simulink model "bcccc"  (Simulink 7.4)
settings: Solver=ode1  StartTime=0.0  StopTime=1000  FixedStep=T  RelTol=1e-3  AbsTol=1e-6
values from neighbouring files (symbols this model uses):
  calibParams = [469.5 7.95034094731e-05 741.8 8.4355330608e-05 2167.3 0.000136518771331]    [bcc.mat]    (also in calibParams.mat = [471.3 8.26262433661e-05 786 8.69187309865e-05 2173.5 0.0001)
  T = 0.5    [bcc.mat]    (also in hydrostart.m = 0.25)
libraries: hydro2pumps_lib x1, simulink_extras x1
settings Model: Creator=dmedonza  LastModifiedBy=student
settings DataIOCC: LimitDataPoints=off  SignalLoggingName=sigsOut
settings OptimizationCC: BooleanDataType=off
settings DebuggingCC: SaveWithParameterizedLinksMsg=none  SignalResolutionControl=TryResolveAllWithWarning  SolverPrmCheckMsg=none  MultiTaskDSMMsg=warning  MultiTaskCondExecSysMsg=none  StrictBusMsg=None
settings HardwareCC: TargetUnknown=on
settings RTWCC: TemplateMakefile=grt_vc.tmf  IncludeERTFirstTime=on

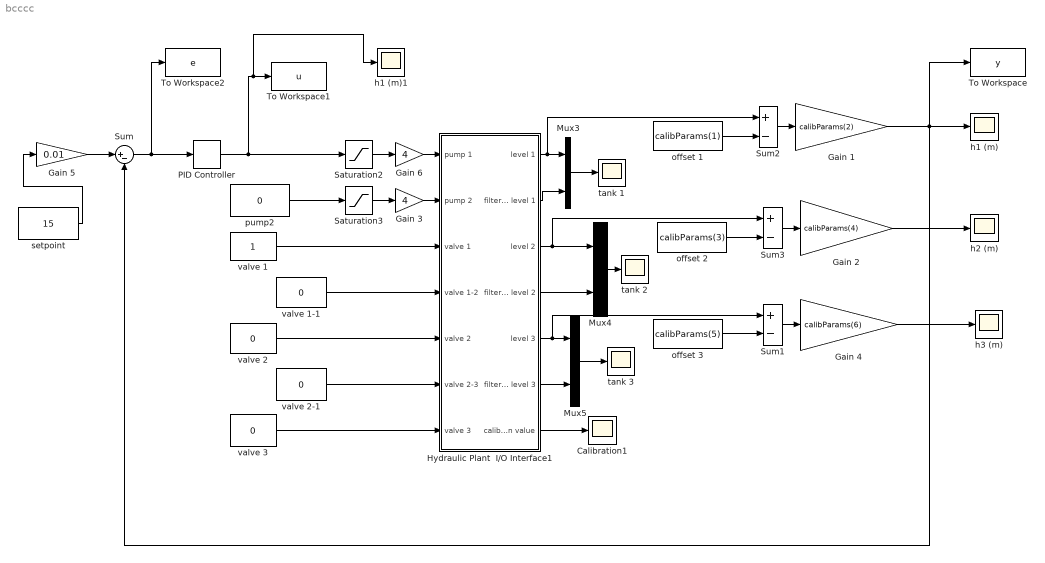
== system bcccc ==
  Calibration1 : Scope
      settings: TickLabels=on  TimeRange=20  YMin=0  YMax=100  SaveName=l  DataFormat=Array
  Gain 1 : Gain  Gain=calibParams(2)  ParameterDataType=sfix(16)  ParameterScaling=2^0  OutDataType=sfix(16)  OutScaling=2^0  SaturateOnIntegerOverflow=on  OutDataTypeStr=Inherit: Same as input  ParamDataTypeStr=Inherit: Same as input
  Gain 2 : Gain  Gain=calibParams(4)  ParameterDataType=sfix(16)  ParameterScaling=2^0  OutDataType=sfix(16)  OutScaling=2^0  SaturateOnIntegerOverflow=on  OutDataTypeStr=Inherit: Same as input  ParamDataTypeStr=Inherit: Same as input
  Gain 3 : Gain  Gain=4  ParameterDataType=sfix(16)  ParameterScaling=2^0  OutDataType=sfix(16)  OutScaling=2^0  SaturateOnIntegerOverflow=on  OutDataTypeStr=Inherit: Same as input  ParamDataTypeStr=Inherit: Same as input
  Gain 4 : Gain  Gain=calibParams(6)  ParameterDataType=sfix(16)  ParameterScaling=2^0  OutDataType=sfix(16)  OutScaling=2^0  SaturateOnIntegerOverflow=on  OutDataTypeStr=Inherit: Same as input  ParamDataTypeStr=Inherit: Same as input
  Gain 5 : Gain  Gain=0.01  ParameterDataType=sfix(16)  ParameterScaling=2^0  OutDataType=sfix(16)  OutScaling=2^0  SaturateOnIntegerOverflow=on  OutDataTypeStr=Inherit: Same as input  ParamDataTypeStr=Inherit: Same as input
  Gain 6 : Gain  Gain=4  ParameterDataType=sfix(16)  ParameterScaling=2^0  OutDataType=sfix(16)  OutScaling=2^0  SaturateOnIntegerOverflow=on  OutDataTypeStr=Inherit: Same as input  ParamDataTypeStr=Inherit: Same as input
  Hydraulic Plant  I/O Interface1 : Subsystem
      mask Display: disp('Two Pumps\nHydraulic\nPlant\nI/O Interface')
  Mux3 : Mux  Inputs=2
  Mux4 : Mux  Inputs=2
  Mux5 : Mux  Inputs=2
  PID Controller : simulink_extras/Additional Linear/PID Controller  SystemSampleTime=-1  P=24*9.9823  I=9.9823  D=0
  Saturation2 : Saturate  UpperLimit=100  LowerLimit=0
  Saturation3 : Saturate  UpperLimit=100  LowerLimit=0
  Sum : Sum  Inputs=|+-  OutDataType=fixdt(1, 16)  OutScaling=2^0
  Sum1 : Sum  Inputs=+-  OutDataType=sfix(16)  OutScaling=2^0  SaturateOnIntegerOverflow=on
  Sum2 : Sum  Inputs=+-  OutDataType=sfix(16)  OutScaling=2^0  SaturateOnIntegerOverflow=on
  Sum3 : Sum  Inputs=+-  OutDataType=sfix(16)  OutScaling=2^0  SaturateOnIntegerOverflow=on
  To Workspace : ToWorkspace  VariableName=y  SampleTime=-1  SaveFormat=Structure
  To Workspace1 : ToWorkspace  VariableName=u  SampleTime=-1  SaveFormat=Structure
  To Workspace2 : ToWorkspace  VariableName=e  SampleTime=-1  SaveFormat=Structure
  h1 (m) : Scope
      settings: TickLabels=on  TimeRange=60  YMin=0.1462  YMax=0.148  SaveName=level1  DataFormat=Array
  h1 (m)1 : Scope
      settings: TickLabels=on  TimeRange=60  YMin=0.1462  YMax=0.148  SaveName=level  DataFormat=Array
  h2 (m) : Scope
      settings: TickLabels=on  TimeRange=60  YMin=0.2499  YMax=0.250425  SaveName=level2  DataFormat=Array
  h3 (m) : Scope
      settings: TickLabels=on  TimeRange=60  YMin=0.2561  YMax=0.2571  SaveName=level3  DataFormat=Array
  offset 1 : Constant  Value=calibParams(1)  OutDataType=sfix(16)  OutScaling=2^0
  offset 2 : Constant  Value=calibParams(3)  OutDataType=sfix(16)  OutScaling=2^0
  offset 3 : Constant  Value=calibParams(5)  OutDataType=sfix(16)  OutScaling=2^0
  pump2 : Constant  Value=0  OutDataType=sfix(16)  OutScaling=2^0
  setpoint : Constant  Value=15  OutDataType=sfix(16)  OutScaling=2^0
  tank 1 : Scope
      settings: TickLabels=on  TimeRange=10  YMin=478  YMax=482  SaveName=tank1  DataFormat=Array  SampleInput=on
  tank 2 : Scope
      settings: TickLabels=on  TimeRange=20  YMin=762.5  YMax=820  SaveName=tank2  DataFormat=Array  SampleInput=on
  tank 3 : Scope
      settings: TickLabels=on  TimeRange=10  YMin=685  YMax=690  SaveName=tank3  DataFormat=Array  SampleInput=on
  valve 1 : Constant  OutDataType=sfix(16)  OutScaling=2^0
  valve 1-1 : Constant  Value=0  OutDataType=sfix(16)  OutScaling=2^0
  valve 2 : Constant  Value=0  OutDataType=sfix(16)  OutScaling=2^0
  valve 2-1 : Constant  Value=0  OutDataType=sfix(16)  OutScaling=2^0
  valve 3 : Constant  Value=0  OutDataType=sfix(16)  OutScaling=2^0
  wires:
  Mux3/1 -> tank 1/1
  Mux5/1 -> tank 3/1
  valve 1/1 -> Hydraulic Plant  I/O Interface1/3(valve 1)
  valve 1-1/1 -> Hydraulic Plant  I/O Interface1/4(valve 1-2)
  valve 2/1 -> Hydraulic Plant  I/O Interface1/5(valve 2)
  valve 2-1/1 -> Hydraulic Plant  I/O Interface1/6(valve 2-3)
  valve 3/1 -> Hydraulic Plant  I/O Interface1/7(valve 3)
  Hydraulic Plant  I/O Interface1/1(level 1) -> Mux3/1, Sum2/1
  Hydraulic Plant  I/O Interface1/2(filtered level 1) -> Mux3/2
  Hydraulic Plant  I/O Interface1/3(level 2) -> Mux4/1, Sum3/1
  Hydraulic Plant  I/O Interface1/4(filtered level 2) -> Mux4/2
  Hydraulic Plant  I/O Interface1/5(level 3) -> Mux5/1, Sum1/1
  Hydraulic Plant  I/O Interface1/6(filtered level 3) -> Mux5/2
  Hydraulic Plant  I/O Interface1/7(calibration value) -> Calibration1/1
  Mux4/1 -> tank 2/1
  offset 1/1 -> Sum2/2
  Sum2/1 -> Gain 1/1
  Gain 6/1 -> Hydraulic Plant  I/O Interface1/1(pump 1)
  Gain 3/1 -> Hydraulic Plant  I/O Interface1/2(pump 2)
  Saturation2/1 -> Gain 6/1
  Saturation3/1 -> Gain 3/1
  offset 2/1 -> Sum3/2
  Sum3/1 -> Gain 2/1
  PID Controller/1 -> Saturation2/1, To Workspace1/1, h1 (m)1/1
  pump2/1 -> Saturation3/1
  Gain 1/1 -> h1 (m)/1, Sum/2, To Workspace/1
  Gain 2/1 -> h2 (m)/1
  offset 3/1 -> Sum1/2
  Sum1/1 -> Gain 4/1
  Gain 4/1 -> h3 (m)/1
  Sum/1 -> PID Controller/1, To Workspace2/1
  setpoint/1 -> Gain 5/1
  Gain 5/1 -> Sum/1

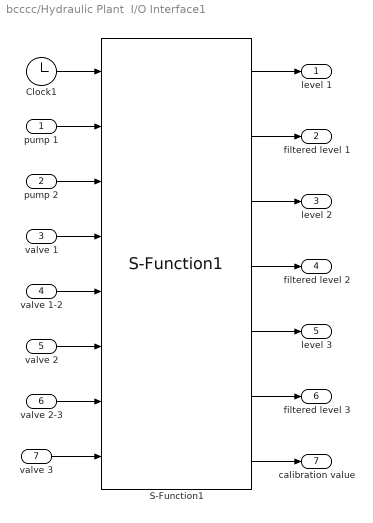
== system bcccc/Hydraulic Plant  I/O Interface1 ==
  pump 1 : Inport  OutDataType=sfix(16)  OutScaling=2^0
  pump 2 : Inport  Port=2  OutDataType=sfix(16)  OutScaling=2^0
  valve 1 : Inport  Port=3  OutDataType=sfix(16)  OutScaling=2^0
  valve 1-2 : Inport  Port=4  OutDataType=sfix(16)  OutScaling=2^0
  valve 2 : Inport  Port=5  OutDataType=sfix(16)  OutScaling=2^0
  valve 2-3 : Inport  Port=6  OutDataType=sfix(16)  OutScaling=2^0
  valve 3 : Inport  Port=7  OutDataType=sfix(16)  OutScaling=2^0
  Clock1 : Clock
      settings: Decimation=10
  S-Function1 : hydro2pumps_lib/S-Function1  Priority=1  com_port=COM4  Ts=T  events_ot=2  rd_timeout=125  matlab_prior=ABOVE_NORMAL_PRIORITY  warning=on  printout=off
  level 1 : Outport
  filtered level 1 : Outport  Port=2
  level 2 : Outport  Port=3
  filtered level 2 : Outport  Port=4
  level 3 : Outport  Port=5
  filtered level 3 : Outport  Port=6
  calibration value : Outport  Port=7
  wires:
  S-Function1/1 -> level 1/1
  S-Function1/2 -> filtered level 1/1
  Clock1/1 -> S-Function1/1
  pump 1/1 -> S-Function1/2
  pump 2/1 -> S-Function1/3
  S-Function1/3 -> level 2/1
  S-Function1/4 -> filtered level 2/1
  S-Function1/5 -> level 3/1
  S-Function1/6 -> filtered level 3/1
  valve 1/1 -> S-Function1/4
  valve 1-2/1 -> S-Function1/5
  valve 2/1 -> S-Function1/6
  valve 2-3/1 -> S-Function1/7
  S-Function1/7 -> calibration value/1
  valve 3/1 -> S-Function1/8
